simulink model "awning_chart"  (R2022a)
settings: Solver=FixedStepDiscrete  StartTime=0.0  StopTime=10.0  FixedStep=0.1  RelTol=1e-3  EnableMultiTasking=on
settings Model: Creator=Amin  LastModifiedBy=Amin
settings SolverCC: AlgebraicLoopSolver=TrustRegion  AutoInsertRateTranBlk=on
settings DataIOCC: LimitDataPoints=on
settings OptimizationCC: DefaultParameterBehavior=Inlined  EnhancedBackFolding=on  PassReuseOutputArgsAs=Individual arguments  ZeroExternalMemoryAtStartup=off  ZeroInternalMemoryAtStartup=off  OptimizeBlockOrder=speed  DifferentSizesBufferReuse=on  OptimizationCustomize=off  EfficientTunableParamExpr=on
settings DebuggingCC: ParameterTunabilityLossMsg=error  UnconnectedInputMsg=warning  UnconnectedOutputMsg=warning  UnconnectedLineMsg=warning  AllowSymbolicDim=off  SFUnexpectedBacktrackingDiag=warning  SFNoUnconditionalDefaultTransitionDiag=warning  SFExecutionAtInitializationDiag=none  ArithmeticOperatorsInVariantConditions=warning
settings SFSimCC: SimUseLocalCustomCode=off  MATLABDynamicMemAlloc=off  CustomCodeUndefinedFunction=UseInterfaceOnly
settings RTWCC: SystemTargetFile=ert.tlc  TemplateMakefile=ert_default_tmf  RTWUseLocalCustomCode=off  DLArmComputeVersion=19.05
settings CodeAppCC: ForceParamTrailComments=on  IgnoreCustomStorageClasses=off  OperatorAnnotations=on  SimulinkDataObjDesc=on  SFDataObjDesc=on  InsertBlockDesc=on
settings ERTTargetCC: GenerateSampleERTMain=on  InlinedParameterPlacement=NonHierarchical  ERTCustomFileTemplate=example_file_process.tlc
settings ConfigComp: CovMetricSettings=dw  CovSaveCumulativeToWorkspaceVar=on  CovSaveSingleToWorkspaceVar=on  CovExternalEMLEnable=off  CovSFcnEnable=off

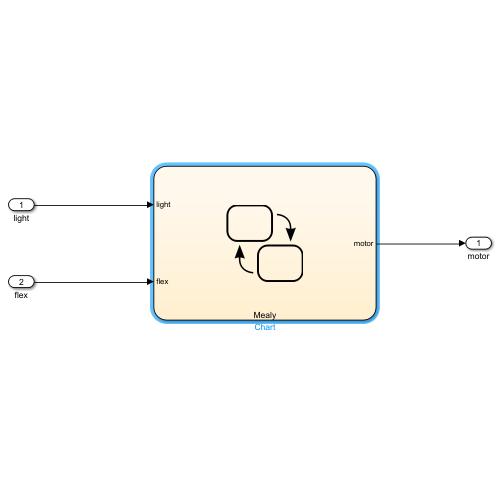
[thumbnail: Simulink's stored preview of the top-level diagram]
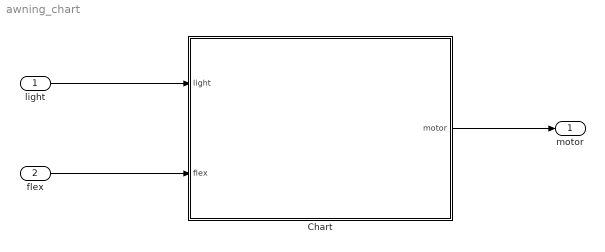
== system awning_chart ==
  light : Inport
  flex : Inport  Port=2
  Chart : Stateflow chart  TreatAsAtomicUnit=on
  motor : Outport
  wires:
  Chart/1(motor) -> motor/1
  light/1 -> Chart/1(light)
  flex/1 -> Chart/2(flex)

== stateflow chart awning_chart/Chart ==
  settings: stateMachineType=MEALY_MACHINE
  state Opening
  state Off
  state Closing
  Off -> Opening [order 1] : [light<45 && flex>10 && flex<80]{motor=1}
  Opening -> Opening [order 3] : {motor=1}
  Opening -> Off [order 1] : [(light>=45 && light<=55) || flex<=10 || flex>=80]{motor=0}
  Opening -> Closing [order 2] : [light>55 && flex>10 && flex<80]{motor=-1}
  Closing -> Opening [order 2] : [light<45 && flex>10 && flex<80]{motor=1}
  (default) -> Off
  Off -> Off [order 3] : {motor=0}
  Off -> Closing [order 2] : [light>55 && flex>10 && flex<80]{motor=-1}
  Closing -> Off [order 1] : [(light>=45 && light<=55) || flex<=10 || flex>=80]{motor=0}
  Closing -> Closing [order 3] : {motor=-1}
  data: motor output; light input; flex input
